simulink model "PMSMmotor_exercise_version"  (Simulink 8.2)
settings: Solver=ode45  StartTime=0  StopTime=2  FixedStep=1/fs/4  MaxStep=1/fs  RelTol=1e-7
InitFcn:
  | Motor_parameters_Lsrpm7fw
values from neighbouring files (symbols this model uses):
  fs = 10e3    (= 10000)    [Motor_parameters_Lsrpm7fw.m]
  J = 1*1e-3    (= 0.001)    [Motor_parameters_Lsrpm7fw.m]
  Ld = 10e-3    (= 0.01)    [Motor_parameters_Lsrpm7fw.m]
  Lndd_ini = Lndmpm    (= 0.412)    [Motor_parameters_Lsrpm7fw.m]
  Lndmpm = 0.412*1    (= 0.412)    [Motor_parameters_Lsrpm7fw.m]
  Lq = 12.8e-3    (= 0.0128)    [Motor_parameters_Lsrpm7fw.m]
  Npp = 8/2    (= 4)    [Motor_parameters_Lsrpm7fw.m]
  Omegae = 2*pi*5    (= 31.4159265359)    [Motor_parameters_Lsrpm7fw.m]
  Rs = 0.78    [Motor_parameters_Lsrpm7fw.m]
undefined symbols (not defined in the file or in its folder): dfilt, sigbuilder_block
libraries: dsparch4 x3, simulink x1
settings Model: Creator=klu  LastModifiedBy=Fitim k
settings OptimizationCC: BooleanDataType=off  InitFltsAndDblsToZero=on
settings DebuggingCC: AlgebraicLoopMsg=none  SaveWithParameterizedLinksMsg=none  SignalResolutionControl=TryResolveAllWithWarning  SolverPrmCheckMsg=none  MultiTaskDSMMsg=warning  MultiTaskCondExecSysMsg=none
settings RTWCC: IncludeERTFirstTime=on
settings GRTTargetCC: TargetFcnLib=ansi_tfl_tmw.mat

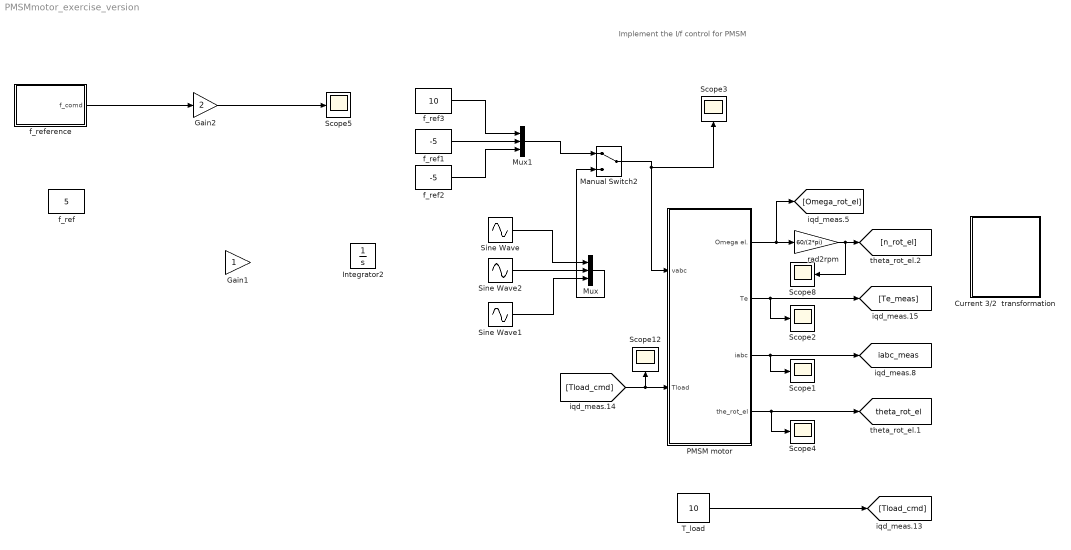
== system PMSMmotor_exercise_version ==
  note: Implement the I/f control for PMSM
  Current 3/2  transformation : Subsystem
      mask Display:
      | plot([0.1000    0.1357    0.1714    0.2071    0.2429    0.2786    0.3143    0.3500    0.3857    0.4214 0.4571    0.4929    0.5286    0.5643    0.6000]-0.05,0.4+0.6*[0.5000    0.5868    0.6564    0.6950    0.6950    0.6564    0.5868    0.5000    0.4132    0.3436 0.3050    0.3050    0.3436    0.4132    0.5000])
      | 
      | plot([0.1,0.9],[0.1,0.9])
      | 
      | plot([0.5,0.9],0.3*[1 1])
  Gain1 : Gain
  Gain2 : Gain  Gain=2
  Integrator2 : Integrator  ExternalReset=rising  LimitOutput=on  UpperSaturationLimit=2
  Manual Switch2 : ManualSwitch
  Mux : Mux  Inputs=3
  Mux1 : Mux  Inputs=3
  PMSM motor : Subsystem
  Scope{1..5,8,12} (7 alike) : Scope
      Scope1 settings: TimeRange=0.09507640067911714  YMin=-4e+51  YMax=7e+51  SaveName=ScopeData22
      Scope12 settings: YMin=0.1  YMax=1.2  SaveName=ScopeData16
      Scope2 settings: TimeRange=3  YMin=-10  YMax=80  SaveName=ScopeData4
      Scope3 settings: YMin=0.1  YMax=1.2  SaveName=ScopeData2
      Scope4 settings: TimeRange=0.09507640067911714  YMin=3  YMax=6.25
      Scope5 settings: TimeRange=2  YMin=1  YMax=13  SaveName=ScopeData8
      Scope8 settings: TimeRange=0.09507640067911714  YMin=285  YMax=315  SaveName=ScopeData23
  Sine Wave : Sin  Amplitude=20  Frequency=Omegae  Phase=pi/2  SampleTime=0
  Sine Wave1 : Sin  Amplitude=20  Frequency=Omegae  Phase=pi/2+2*pi/3  SampleTime=0
  Sine Wave2 : Sin  Amplitude=20  Frequency=Omegae  Phase=pi/2-2*pi/3  SampleTime=0
  T_load : Constant  Value=10
  f_ref : Constant  Value=5
  f_ref1 : Constant  Value=-5
  f_ref2 : Constant  Value=-5
  f_ref3 : Constant  Value=10
  f_reference : Subsystem  Tag=STV Subsys  LoadFcn=sigbuilder_block('load');  StartFcn=sigbuilder_block('start');  StopFcn=sigbuilder_block('stop');  ClipboardFcn=sigbuilder_block('clipboard');  mask(Sigbuilder block){}
      mask help: Simulink:masks:SigbuilderBlock_MD
      mask init:
      | if ~strcmp(get_param(bdroot(gcbh),'SimulationStatus'),'stopped') tuvar = sigbuilder_block('maskInit'); end
      settings: CopyFcn=sigbuilder_block('copy');  DeleteFcn=sigbuilder_block('delete');  ModelCloseFcn=sigbuilder_block('modelClose');  PreSaveFcn=sigbuilder_block('preSave');  PauseFcn=sigbuilder_block('pause');  ContinueFcn=sigbuilder_block('continue');  NameChangeFcn=sigbuilder_block('namechange');  OpenFcn=sigbuilder_block('open',[436.966 199.862 550.552 399.724 ]);  CloseFcn=sigbuilder_block('close');
      mask Display: plot(0, 0, 100, 100,[2, 2, 32, 32, 2], [68, 8, 8, 68, 68],[32, 2], [38, 38], [32, 19, 2],[53, 60, 44], [32, 17, 17, 2],[16, 16, 31, 31]);txt = getActiveGroup(gcbh);text(2, 100, txt,'verticalAlignment', 'top');
  rad2rpm : Gain  Gain=60/(2*pi)
  tag scope: iabc_meas=global, theta_rot_el=global
  wires:
  [Tload_cmd] -> PMSM motor/2(Tload), Scope12/1
  PMSM motor/2(Te) -> Scope2/1, [Te_meas]
  PMSM motor/1(Omega el.) -> [Omega_rot_el], rad2rpm/1
  PMSM motor/3(iabc) -> [iabc_meas], Scope1/1
  PMSM motor/4(the_rot_el) -> [theta_rot_el], Scope4/1
  T_load/1 -> [Tload_cmd]
  rad2rpm/1 -> Scope8/1, [n_rot_el]
  Sine Wave/1 -> Mux/1
  Sine Wave2/1 -> Mux/2
  Sine Wave1/1 -> Mux/3
  Mux/1 -> Manual Switch2/2
  Mux1/1 -> Manual Switch2/1
  f_ref3/1 -> Mux1/1
  f_ref1/1 -> Mux1/2
  f_ref2/1 -> Mux1/3
  Manual Switch2/1 -> Scope3/1, PMSM motor/1(vabc)
  Gain2/1 -> Scope5/1
  f_reference/1(f_comd) -> Gain2/1

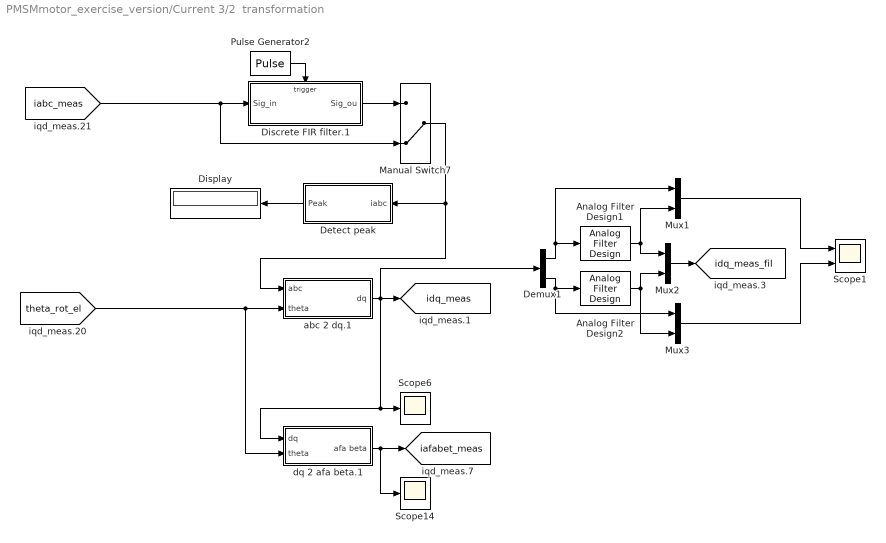
== system PMSMmotor_exercise_version/Current 3/2  transformation ==
  Analog Filter Design1 : dsparch4/Analog Filter Design  method=Butterworth  filttype=Lowpass  N=5  Wlo=2*pi*400  Whi=80  Rp=2  Rs=40
  Analog Filter Design2 : dsparch4/Analog Filter Design  method=Butterworth  filttype=Lowpass  N=5  Wlo=2*pi*400  Whi=80  Rp=2  Rs=40
  Demux1 : Demux  Outputs=2
  Detect peak : Subsystem
  Discrete FIR filter.1 : Subsystem
  Display : Display
  Manual Switch7 : ManualSwitch  CurrentSetting=0
  Mux1 : Mux  Inputs=2
  Mux2 : Mux  Inputs=2
  Mux3 : Mux  Inputs=2
  Pulse Generator2 : DiscretePulseGenerator  PulseType=Time based  Period=1/fs  PulseWidth=50  PhaseDelay=1/fs/4*0
  Scope1 : Scope  NumInputPorts=2
      settings: YMin=-5500~-5  YMax=5500~5  SaveName=ScopeData40
  Scope14 : Scope
      settings: YMin=-5500  YMax=5500  SaveName=ScopeData27
  Scope6 : Scope
      settings: SaveName=ScopeData25
  abc 2 dq.1 : Subsystem
  dq 2 afa beta.1 : Subsystem
  tag scope: iafabet_meas=global, idq_meas=global, idq_meas_fil=global
  wires:
  abc 2 dq.1/1(dq) -> [idq_meas], Demux1/1, Scope6/1, dq 2 afa beta.1/1(dq)
  dq 2 afa beta.1/1(afa beta) -> [iafabet_meas], Scope14/1
  Pulse Generator2/1 -> Discrete FIR filter.1/Trigger
  Manual Switch7/1 -> abc 2 dq.1/1(abc), Detect peak/1(iabc)
  [iabc_meas] -> Discrete FIR filter.1/1(Sig_in), Manual Switch7/2
  Discrete FIR filter.1/1(Sig_ou) -> Manual Switch7/1
  Detect peak/1(Peak) -> Display/1
  [theta_rot_el] -> abc 2 dq.1/2(theta), dq 2 afa beta.1/2(theta)
  Demux1/1 -> Analog Filter Design1/1, Mux1/1
  Demux1/2 -> Analog Filter Design2/1, Mux3/1
  Analog Filter Design1/1 -> Mux2/1, Mux1/2
  Analog Filter Design2/1 -> Mux2/2, Mux3/2
  Mux1/1 -> Scope1/1
  Mux3/1 -> Scope1/2
  Mux2/1 -> [idq_meas_fil]

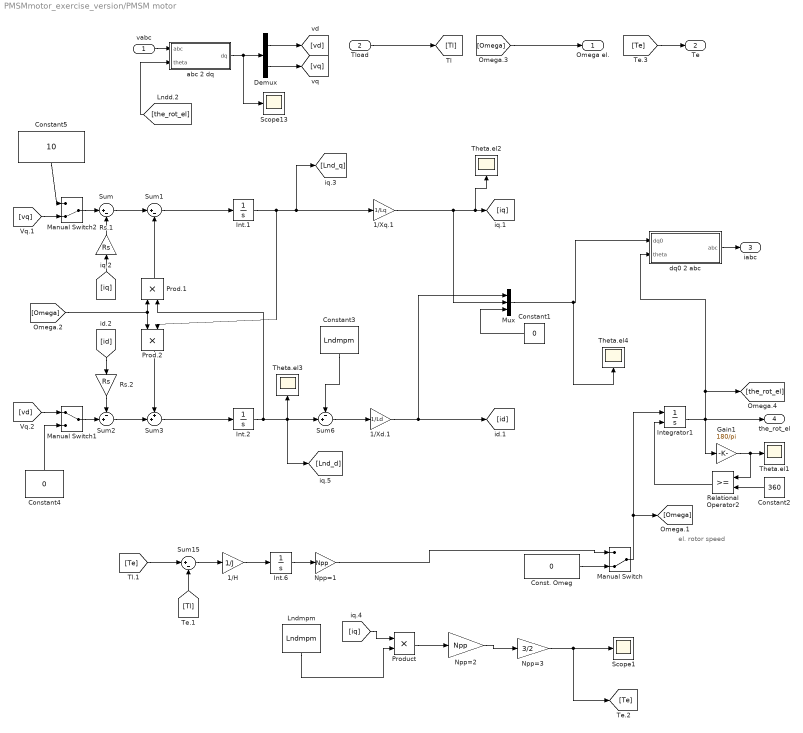
== system PMSMmotor_exercise_version/PMSM motor ==
  note: el. rotor speed
  vabc : Inport
  Tload : Inport  Port=2
  1/H : Gain  Gain=1/J
  1/Xd.1 : Gain  Gain=1/Ld
  1/Xq.1 : Gain  Gain=1/Lq
  Const. Omeg : Constant  Value=0
  Constant1 : Constant  Value=0
  Constant2 : Constant  Value=360
  Constant3 : Constant  Value=Lndmpm
  Constant4 : Constant  Value=0
  Constant5 : Constant  Value=10
  Demux : Demux  Outputs=2
  Gain1 : Gain  Gain=180/pi
  Int.1 : Integrator
  Int.2 : Integrator  InitialCondition=Lndd_ini
  Int.6 : Integrator  InitialCondition=1
  Integrator1 : Integrator  ExternalReset=rising
  Lndmpm : Constant  Value=Lndmpm
  Manual Switch : ManualSwitch  CurrentSetting=0
  Manual Switch1 : ManualSwitch
  Manual Switch2 : ManualSwitch  CurrentSetting=0
  Mux : Mux  Inputs=3
  Npp=1 : Gain  Gain=Npp
  Npp=2 : Gain  Gain=Npp
  Npp=3 : Gain  Gain=3/2
  Prod.1 : Product  RndMeth=Zero
  Prod.2 : Product  RndMeth=Zero
  Product : Product  RndMeth=Zero
  Relational Operator2 : RelationalOperator  OutDataTypeStr=boolean
  Rs.1 : Gain  Gain=Rs
  Rs.2 : Gain  Gain=Rs
  Scope1 : Scope
      settings: TimeRange=2  YMin=-1  YMax=21  SaveName=ScopeData3
  Scope13 : Scope
      settings: TimeRange=2  YMin=-1  YMax=21  SaveName=ScopeData24
  Sum : Sum  Inputs=|+-
  Sum1 : Sum  Inputs=|+-
  Sum15 : Sum  Inputs=|+-
  Sum2 : Sum  Inputs=-+|
  Sum3 : Sum  Inputs=++|
  Sum6 : Sum  Inputs=-+|
  Theta.el{1..4} (4 alike) : Scope
      Theta.el1 settings: YMin=-225  YMax=225
      Theta.el2 settings: YMin=-225  YMax=225  SaveName=ScopeData5
      Theta.el3 settings: YMin=-225  YMax=225  SaveName=ScopeData6
      Theta.el4 settings: YMin=-225  YMax=225  SaveName=ScopeData7
  abc 2 dq : Subsystem
  dq0 2 abc : Subsystem
  Omega el. : Outport
  Te : Outport  Port=2
  iabc : Outport  Port=3
  the_rot_el : Outport  Port=4
  wires:
  [Omega] -> Omega el./1
  [Te] -> Te/1
  Tload/1 -> [Tl]
  Demux/2 -> [vq]
  Demux/1 -> [vd]
  dq0 2 abc/1(abc) -> iabc/1
  Integrator1/1 -> Gain1/1, the_rot_el/1, dq0 2 abc/2(theta), [the_rot_el]
  Gain1/1 -> Theta.el1/1, Relational Operator2/1
  Constant2/1 -> Relational Operator2/2
  Relational Operator2/1 -> Integrator1/2
  vabc/1 -> abc 2 dq/1(abc)
  abc 2 dq/1(dq) -> Demux/1, Scope13/1
  [the_rot_el] -> abc 2 dq/2(theta)
  Const. Omeg/1 -> Manual Switch/2
  Manual Switch/1 -> [Omega], Integrator1/1
  Rs.1/1 -> Sum/2
  Sum/1 -> Sum1/1
  Int.1/1 -> [Lnd_q], 1/Xq.1/1, Prod.2/2
  1/Xq.1/1 -> Mux/2, Theta.el2/1, [iq]
  [iq] -> Rs.1/1
  1/Xd.1/1 -> Mux/1, [id]
  Rs.2/1 -> Sum2/1
  [id] -> Rs.2/1
  Sum2/1 -> Sum3/2
  [Omega] -> Prod.1/1, Prod.2/1
  Sum1/1 -> Int.1/1
  Sum3/1 -> Int.2/1
  Mux/1 -> Theta.el4/1, dq0 2 abc/1(dq0)
  Prod.1/1 -> Sum1/2
  Prod.2/1 -> Sum3/1
  [Te] -> Sum15/1
  Sum15/1 -> 1/H/1
  1/H/1 -> Int.6/1
  Int.6/1 -> Npp=1/1
  Npp=1/1 -> Manual Switch/1
  [Tl] -> Sum15/2
  Int.2/1 -> Theta.el3/1, [Lnd_d], Sum6/2, Prod.1/2
  Constant1/1 -> Mux/3
  Sum6/1 -> 1/Xd.1/1
  Constant3/1 -> Sum6/1
  [iq] -> Product/1
  Lndmpm/1 -> Product/2
  Product/1 -> Npp=2/1
  Npp=3/1 -> Scope1/1, [Te]
  Npp=2/1 -> Npp=3/1
  Manual Switch1/1 -> Sum2/2
  [vd] -> Manual Switch1/1
  Constant4/1 -> Manual Switch1/2
  Manual Switch2/1 -> Sum/1
  [vq] -> Manual Switch2/2
  Constant5/1 -> Manual Switch2/1

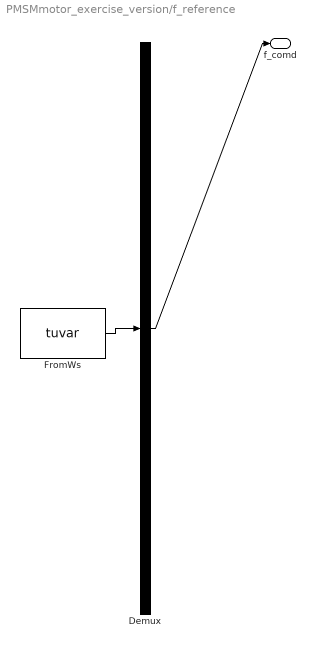
== system PMSMmotor_exercise_version/f_reference ==
  Demux : Demux  Tag=STV Demux  Outputs=1
  FromWs : FromWorkspace  Tag=STV FromWs  VariableName=tuvar  SampleTime=0  SigBuilderData=DataTag1  VnvData=DataTag2
      SigBuilderData=|
      | common.afterFinalStr = 'Extrapolate'
      | common.sampleTime = 0
      | dataSet.timeRange = [0 10]
      | dataSet.name = 'Group 1'
      | sbobj.Groups.Name = 'Group 1'
      | sbobj.Groups.Signals.Name = 'f_comd'
      | sbobj.Groups.Signals.XData = [0 1 2 10]
      | sbobj.Groups.Signals.YData = [0 1 1 1]
  f_comd : Outport  Tag=STV Outport
  wires:
  FromWs/1 -> Demux/1
  Demux/1 -> f_comd/1

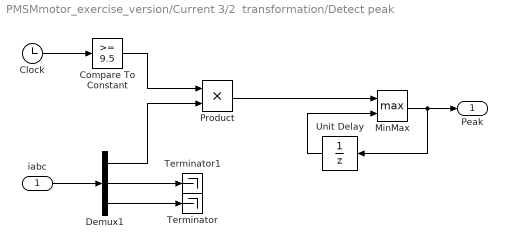
== system PMSMmotor_exercise_version/Current 3/2  transformation/Detect peak ==
  iabc : Inport
  Clock : Clock
  Compare To Constant : simulink/Logic and Bit Operations/Compare To Constant  relop=>=  const=9.5  OutDataTypeStr=uint8  ZeroCross=off
  Demux1 : Demux  Outputs=3
  MinMax : MinMax  Function=max  Inputs=2
  Product : Product  RndMeth=Zero
  Terminator : Terminator
  Terminator1 : Terminator
  Unit Delay : UnitDelay  SampleTime=1/5e3
  Peak : Outport
  wires:
  iabc/1 -> Demux1/1
  Demux1/3 -> Terminator/1
  Demux1/2 -> Terminator1/1
  Clock/1 -> Compare To Constant/1
  Compare To Constant/1 -> Product/1
  Demux1/1 -> Product/2
  MinMax/1 -> Peak/1, Unit Delay/1
  Product/1 -> MinMax/1
  Unit Delay/1 -> MinMax/2

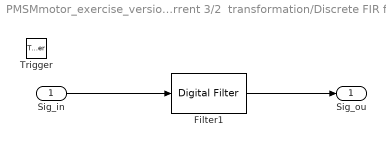
== system PMSMmotor_exercise_version/Current 3/2  transformation/Discrete FIR filter.1 ==
  Sig_in : Inport
  Trigger : TriggerPort
  Filter1 : dsparch4/Digital Filter  Tag=BlockMethodSubSystem  TypePopup=FIR (all zeros)  IIRFiltStruct=Direct form II transposed  AllPoleFiltStruct=Direct form  FIRFiltStruct=Direct form  CoeffSource=Specify via dialog  NumCoeffs=[0.0129982054114534 -0.101337899103369 0.58834244300993 0.58834244300993 -0.101337899103369 0.0129982054114534]  DenCoeffs=[1 0.1]  BiQuadCoeffs=[1 0.3 0.4 1 0.1 0.2]  LatticeCoeffs=[0.2 0.4]  denIgnore=on  FiltPerSampPopup=One filter per frame  IC=0  ICnum=0  ICden=0  roundingMode=Floor  overflowMode=off  ScaleValues=1  scaleValueFracLength=14  stageInFracLength=15  stageOutFracLength=15  FilterSource=Specify via dialog  dfiltObjectName=dfilt.dffir([1 2 1])  InputProcessing=Inherited (this choice will be removed - see release notes)
  Sig_ou : Outport
  wires:
  Sig_in/1 -> Filter1/1
  Filter1/1 -> Sig_ou/1

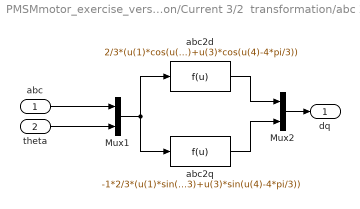
== system PMSMmotor_exercise_version/Current 3/2  transformation/abc 2 dq.1 ==
  abc : Inport
  theta : Inport  Port=2
  Mux1 : Mux  Inputs=2
  Mux2 : Mux  Inputs=2
  abc2d : Fcn  Expr=2/3*(u(1)*cos(u(4))+u(2)*cos(u(4)-2*pi/3)+u(3)*cos(u(4)-4*pi/3))
  abc2q : Fcn  Expr=-1*2/3*(u(1)*sin(u(4))+u(2)*sin(u(4)-2*pi/3)+u(3)*sin(u(4)-4*pi/3))
  dq : Outport
  wires:
  Mux2/1 -> dq/1
  abc2q/1 -> Mux2/2
  abc2d/1 -> Mux2/1
  Mux1/1 -> abc2q/1, abc2d/1
  theta/1 -> Mux1/2
  abc/1 -> Mux1/1

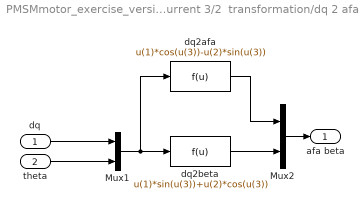
== system PMSMmotor_exercise_version/Current 3/2  transformation/dq 2 afa beta.1 ==
  dq : Inport
  theta : Inport  Port=2
  Mux1 : Mux  Inputs=2
  Mux2 : Mux  Inputs=2
  dq2afa : Fcn  Expr=u(1)*cos(u(3))-u(2)*sin(u(3))
  dq2beta : Fcn  Expr=u(1)*sin(u(3))+u(2)*cos(u(3))
  afa beta : Outport
  wires:
  dq/1 -> Mux1/1
  theta/1 -> Mux1/2
  Mux1/1 -> dq2beta/1, dq2afa/1
  dq2afa/1 -> Mux2/1
  dq2beta/1 -> Mux2/2
  Mux2/1 -> afa beta/1

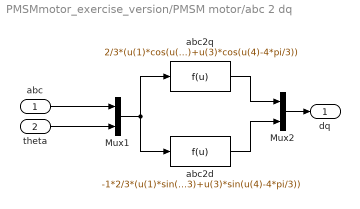
== system PMSMmotor_exercise_version/PMSM motor/abc 2 dq ==
  abc : Inport
  theta : Inport  Port=2
  Mux1 : Mux  Inputs=2
  Mux2 : Mux  Inputs=2
  abc2d : Fcn  Expr=-1*2/3*(u(1)*sin(u(4))+u(2)*sin(u(4)-2*pi/3)+u(3)*sin(u(4)-4*pi/3))
  abc2q : Fcn  Expr=2/3*(u(1)*cos(u(4))+u(2)*cos(u(4)-2*pi/3)+u(3)*cos(u(4)-4*pi/3))
  dq : Outport
  wires:
  Mux2/1 -> dq/1
  abc2d/1 -> Mux2/2
  abc2q/1 -> Mux2/1
  Mux1/1 -> abc2d/1, abc2q/1
  theta/1 -> Mux1/2
  abc/1 -> Mux1/1

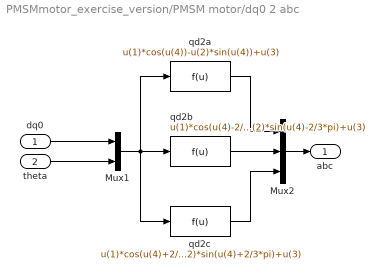
== system PMSMmotor_exercise_version/PMSM motor/dq0 2 abc ==
  dq0 : Inport
  theta : Inport  Port=2
  Mux1 : Mux  Inputs=2
  Mux2 : Mux  Inputs=3
  qd2a : Fcn  Expr=u(1)*cos(u(4))-u(2)*sin(u(4))+u(3)
  qd2b : Fcn  Expr=u(1)*cos(u(4)-2/3*pi)-u(2)*sin(u(4)-2/3*pi)+u(3)
  qd2c : Fcn  Expr=u(1)*cos(u(4)+2/3*pi)-u(2)*sin(u(4)+2/3*pi)+u(3)
  abc : Outport
  wires:
  Mux2/1 -> abc/1
  qd2b/1 -> Mux2/2
  qd2a/1 -> Mux2/1
  Mux1/1 -> qd2b/1, qd2c/1, qd2a/1
  theta/1 -> Mux1/2
  dq0/1 -> Mux1/1
  qd2c/1 -> Mux2/3
